simulink model "D53_LKAS_JLU_20200911_1116"  (R2018b)
settings: Solver=ode3  StartTime=0.0  StopTime=10.0  FixedStep=0.01  RelTol=1e-3  EnableMultiTasking=on
model workspace (MAT data in the model file):
  MCOS : class17 (value not decoded)
  MCOS : class17 (value not decoded)
  MCOS : class17 (value not decoded)
  MCOS : class17 (value not decoded)
  MCOS : class17 (value not decoded)
  MCOS : class17 (value not decoded)
  MCOS : class17 (value not decoded)
  MCOS : class17 (value not decoded)
  MCOS : class17 (value not decoded)
  MCOS : class17 (value not decoded)
  MCOS : class17 (value not decoded)
  MCOS : class17 (value not decoded)
  MCOS : class17 (value not decoded)
  MCOS : class17 (value not decoded)
  MCOS : class17 (value not decoded)
  MCOS : class17 (value not decoded)
  MCOS : class17 (value not decoded)
  MCOS : class17 (value not decoded)
  MCOS : class17 (value not decoded)
  MCOS : class17 (value not decoded)
  MCOS : class17 (value not decoded)
  MCOS : class17 (value not decoded)
  MCOS : class17 (value not decoded)
  MCOS : class17 (value not decoded)
  MCOS : class17 (value not decoded)
  MCOS : class17 (value not decoded)
  MCOS : class17 (value not decoded)
  MCOS : class17 (value not decoded)
  MCOS : class17 (value not decoded)
  MCOS : class17 (value not decoded)
  MCOS : class17 (value not decoded)
  MCOS : class17 (value not decoded)
  MCOS : class17 (value not decoded)
  MCOS : class17 (value not decoded)
  MCOS : class17 (value not decoded)
  MCOS : class17 (value not decoded)
  MCOS : class17 (value not decoded)
  MCOS : class17 (value not decoded)
  MCOS : class17 (value not decoded)
  MCOS : class17 (value not decoded)
  MCOS : class17 (value not decoded)
  MCOS : class17 (value not decoded)
  MCOS : class17 (value not decoded)
  MCOS : class17 (value not decoded)
  MCOS : class17 (value not decoded)
  MCOS : class17 (value not decoded)
  MCOS : class17 (value not decoded)
  MCOS : class17 (value not decoded)
  MCOS : class17 (value not decoded)
  MCOS : class17 (value not decoded)
  MCOS : class17 (value not decoded)
  MCOS : class17 (value not decoded)
  MCOS : class17 (value not decoded)
  MCOS : class17 (value not decoded)
  MCOS : class17 (value not decoded)
  MCOS : class17 (value not decoded)
  MCOS : class17 (value not decoded)
  MCOS : class17 (value not decoded)
  MCOS : class17 (value not decoded)
  MCOS : class17 (value not decoded)
  MCOS : class17 (value not decoded)
  MCOS : class17 (value not decoded)
  MCOS : class17 (value not decoded)
  MCOS : class17 (value not decoded)
  MCOS : class17 (value not decoded)
  MCOS : class17 (value not decoded)
  MCOS : class17 (value not decoded)
  MCOS : class17 (value not decoded)
  MCOS : class17 (value not decoded)
  MCOS : class17 (value not decoded)
  MCOS : class17 (value not decoded)
  MCOS : class17 (value not decoded)
  MCOS : class17 (value not decoded)
  MCOS : class17 (value not decoded)
  MCOS : class17 (value not decoded)
  MCOS : class17 (value not decoded)
  MCOS : class17 (value not decoded)
  MCOS : class17 (value not decoded)
  MCOS : class17 (value not decoded)
  MCOS : class17 (value not decoded)
  MCOS : class17 (value not decoded)
  MCOS : class17 (value not decoded)
  MCOS : class17 (value not decoded)
  MCOS : class17 (value not decoded)
  MCOS : class17 (value not decoded)
  MCOS : class17 (value not decoded)
  MCOS : class17 (value not decoded)
  MCOS : class17 (value not decoded)
  MCOS : class17 (value not decoded)
undefined symbols (not defined in the file): LKA_CarWidth, LKA_SampleTime, LKA_StrRatio_C, LKA_Veh2CamL_C, LKA_Veh2CamW_C, LKA_WhlBaseL_C, LL_CompSWA_C, LL_CrvtPrvwT_C, LL_DesDvt_C, LL_DvtComp_C, LL_DvtPrvwT_C, LL_DvtSpdDet_vDvtSpdMin_C, LL_HdAgExT_C, LL_HdAgPrvwT_C, LL_LAccMax_C, LL_LAccRMax_C, LL_LDW_EarliestWarnLine_C, LL_LDW_LatestWarnLine_C, LL_LDWS_SUPPRESS_HEADING, LL_LFClb_TFC_DiffCtlBalance, LL_LFClb_TFC_DiffCtrlMaxSWA, LL_LFClb_TFC_DiffCtrlRatio, LL_LFClb_TFC_facmGainLutGain1_C, LL_LFClb_TFC_facmGainLutGain2_C, LL_LFClb_TFC_facmIntegRatio, LL_LFClb_TFC_facmKlat_C, LL_LFClb_TFC_FfCtlRatio_C, LL_LFClb_TFC_phiIntegCtlMaxSWA_C, LL_LFClb_TFC_tiKlatPrvwT_C, LL_LFClb_TFC_vGainLutVehSpdLwr_C, LL_LFClb_TFC_vGainLutVehSpdUpr_C, LL_LKA_EarliestWarnLine_C, LL_LKA_LatestWarnLine_C, LL_LKAExPrcs_ExitC0Dvt, LL_LKAExPrcs_ExitC0Swt, LL_LKAExPrcs_tiExitTime1, LL_LKAExPrcs_tiExitTime2, LL_LKAExPrcs_tiExitTime3, LL_LKAS_OUT_OF_CONTROL_LAT_VEL, LL_LKAS_OUT_OF_CONTROL_TTLC, LL_LKASWASyn_M0, LL_LKASWASyn_M1, LL_LKASWASyn_M2, LL_LKASWASyn_M3K, LL_LKASWASyn_SWAaddMax, LL_LKASWASyn_T2, LL_LKASWASyn_tiTrqSwaRtTime, LL_LKASWASyn_tiTrqSwaTime, LL_LKASWASyn_TrqMax, LL_LKASWASyn_TrqSwaAddSwt, LL_LKASWASyn_TrqSwaRateDiff, LL_LSpdCompT_C, LL_lStpLngth_C, LL_MAX_DELAY_EPSSTAR_TIME, LL_MAX_DRIVER_TORQUE_DISABLE, LL_MAX_DRIVER_TORQUE_ENABLE, LL_MAX_LANE_WIDTH_DISABLE, LL_MAX_LANE_WIDTH_ENABLE, LL_MAX_LAT_ACC_DISABLE, LL_MAX_LAT_ACC_ENABLE ... (+30)
libraries: simulink x134, canmsglib x52, dspstat3 x3, simulink_extras x1
(part 3 of 18)

== system D53_LKAS_JLU_20200911_1116/Clb/Calibration3 ==
  In1 : Inport
  In2 : Inport  Port=2
  Data Type Conversion{1..10} (10 alike) : DataTypeConversion  OutDataTypeStr=single
  If1 : If  IfExpression=u1 ==21  ElseIfExpressions=u1==22,u1==23,u1==24,u1==25,u1==26,u1==27,u1==28,u1==29,u1==30  ShowElse=off
  Rate Transition{1..3,5..11} (10 alike) : RateTransition  Deterministic=off  OutPortSampleTime=0.01
  Subsystem2 : Subsystem
  Out1 : Outport
  Out2 : Outport  Port=2
  Out3 : Outport  Port=3
  Out4 : Outport  Port=4
  Out5 : Outport  Port=5
  Out6 : Outport  Port=6
  Out7 : Outport  Port=7
  Out8 : Outport  Port=8
  Out9 : Outport  Port=9
  Out10 : Outport  Port=10
  wires:
  If1/3 -> Subsystem2/3(In3)
  If1/6 -> Subsystem2/6(In6)
  If1/2 -> Subsystem2/2(In2)
  If1/5 -> Subsystem2/5(In5)
  If1/9 -> Subsystem2/9(In9)
  If1/4 -> Subsystem2/4(In4)
  If1/1 -> Subsystem2/1(In1)
  If1/7 -> Subsystem2/7(In7)
  If1/8 -> Subsystem2/8(In8)
  If1/10 -> Subsystem2/10(In10)
  In1/1 -> If1/1
  In2/1 -> Subsystem2/11(In11)
  Data Type Conversion3/1 -> Rate Transition3/1
  Data Type Conversion2/1 -> Rate Transition2/1
  Data Type Conversion10/1 -> Rate Transition11/1
  Data Type Conversion5/1 -> Rate Transition6/1
  Rate Transition6/1 -> Out5/1
  Subsystem2/5(Out5) -> Data Type Conversion5/1
  Subsystem2/6(Out6) -> Data Type Conversion6/1
  Subsystem2/10(Out10) -> Data Type Conversion10/1
  Subsystem2/1(Out1) -> Data Type Conversion1/1
  Subsystem2/9(Out9) -> Data Type Conversion9/1
  Subsystem2/7(Out7) -> Data Type Conversion7/1
  Subsystem2/8(Out8) -> Data Type Conversion8/1
  Subsystem2/3(Out3) -> Data Type Conversion3/1
  Subsystem2/4(Out4) -> Data Type Conversion4/1
  Data Type Conversion4/1 -> Rate Transition5/1
  Data Type Conversion8/1 -> Rate Transition9/1
  Data Type Conversion9/1 -> Rate Transition10/1
  Data Type Conversion7/1 -> Rate Transition8/1
  Rate Transition8/1 -> Out7/1
  Rate Transition1/1 -> Out1/1
  Rate Transition2/1 -> Out2/1
  Rate Transition5/1 -> Out4/1
  Rate Transition10/1 -> Out9/1
  Rate Transition11/1 -> Out10/1
  Rate Transition3/1 -> Out3/1
  Subsystem2/2(Out2) -> Data Type Conversion2/1
  Data Type Conversion6/1 -> Rate Transition7/1
  Rate Transition7/1 -> Out6/1
  Data Type Conversion1/1 -> Rate Transition1/1
  Rate Transition9/1 -> Out8/1

== system D53_LKAS_JLU_20200911_1116/Clb/Subsystem1 ==
  CAN Unpack : canmsglib/CAN Unpack  MsgList=(none)  MsgName=CAN Msg  MsgIDType=Extended (29-bit identifier)  MsgIdentifier=120534787  MsgLength=8  SignalInfo=Serial number$0$8$1$2$1$0$1$0$-Inf$Inf$#index$8$8$1$2$1$0$1$-100$-Inf$Inf$#coefficient$16$32$1$2$1$0$0.000001$-10$-Inf$Inf$#  NSignals=3  IDPort=off  TimestampPort=off  ErrorPort=off  RemotePort=off  LengthPort=off  StatusPort=off  StartBits=str2num('[int32(0);int32(8);int32(16)]')  SignalSizes=str2num('[int32(8);int32(8);int32(32)]')  ByteOrders=str2num('[int32(1);int32(1);int32(1)]')  DataTypes=str2num('[int32(2);int32(2);int32(2)]')  MultiplexTypes=str2num('[int32(1);int32(1);int32(1)]')  MultiplexValues=str2num('[double(0);double(0);double(0)]')  Factors=str2num('[double(1);double(1);double(0.000001)]')  Offsets=str2num('[double(0);double(-100);double(-10)]')  Minimums=str2num('[double(-Inf);double(-Inf);double(-Inf)]')  Maximums=str2num('[double(Inf);double(Inf);double(Inf)]')  ApplyMinMax=off
      settings: SourceProductName=Simulink Real-Time  SourceProductBaseCode=XP
  S-Function2 : S-Function  FunctionName=CAN_Rec_P  Parameters=uint8(Module-1),uint32(ID),uint8(Frameformat-1),uint8(Newflag),uint8(FIFO),double(sampletime)  SFunctionDeploymentMode=off  EnableBusSupport=off  mask(CAN_receive){Module=CAN_0, ID=120534787, Frameformat=Extended (29-bit identifier), Newflag=on, FIFO=off, sampletime=0.01}
      mask prompts: Module "CAN Port:"; ID "CAN Frame ID:"; Frameformat "CAN Frame Format:"; FIFO "Overflow flag"
      mask init:
      | maskdisplay = canrecicon(Module,ID,Frameformat,Newflag,FIFO);
      | set_param(gcb, 'MaskDisplay', maskdisplay);
      mask TypeOptions Module: CAN_0 | CAN_1 | CAN_2 | CAN_3
      mask TypeOptions Frameformat: Standard (11-bit identifier) | Extended (29-bit identifier)
      mask Display: color('blue');text(0.98,0.9,'MPC5675K','horizontalAlignment','right');color('black');text(0.5,0.6,'FlexCAN_0 Receive','horizontalAlignment','center');text(0.5,0.35,'Extended ID:120534787','horizontalAlignment','center');port_label('output',1,'New_Flag');port_label('output',2,'CAN_Msg');
  Out1 : Outport
  Out2 : Outport  Port=2
  Out3 : Outport  Port=3
  wires:
  S-Function2/2 -> CAN Unpack/1
  CAN Unpack/1 -> Out1/1
  CAN Unpack/2 -> Out2/1
  CAN Unpack/3 -> Out3/1

== system D53_LKAS_JLU_20200911_1116/Clb/Subsystem5 ==
  In1 : Inport
  In2 : Inport  Port=2
  Constant : Constant  Value=10
  Data Type Conversion1 : DataTypeConversion  OutDataTypeStr=single
  Data Type Conversion3 : DataTypeConversion  OutDataTypeStr=single
  Divide : Product  Inputs=**
  Fcn : Fcn  Expr=pow(u(1),u(2))
  Mux : Mux  Inputs=2
  Out1 : Outport
  wires:
  Mux/1 -> Fcn/1
  Fcn/1 -> Divide/1
  In2/1 -> Divide/2
  Divide/1 -> Out1/1
  In1/1 -> Data Type Conversion1/1
  Data Type Conversion1/1 -> Mux/2
  Data Type Conversion3/1 -> Mux/1
  Constant/1 -> Data Type Conversion3/1

== system D53_LKAS_JLU_20200911_1116/LL/Fault_Diagnostic ==
  bsInInfo : Inport
  Bus Creator : BusCreator  Inputs=2
  Bus Creator1 : BusCreator  Inputs=12
  Bus Selector3 : BusSelector  OutputSignals=DTC_Indicator.LKAS_BSWDTC_Status
  Bus Selector4 : BusSelector  OutputSignals=bsVehMovInfo.ESC_VehSpd_Valid,bsEPSInfo.EPS_LKA_State,bsEPSInfo.EPS_Error_State,bsEPSInfo.SAS_Clb_State,bsEPSInfo.SAS_Trim_State,bsSWAInfo.SWS_Fault_Code,bsSWAInfo.SAS_In_Status,bsPTState.TCU_ActualGear,bsEPSInfo.EPS_TrqLim_State,bsEPSInfo.EPS_Trq_State,bsVehMovInfo.ESC_LatAcc_Valid,bsVehMovInfo.ESC_YawRate_Valid,bsVehMovInfo.ESC_LonAcc_Valid
  Compare To Constant26 : simulink/Logic and Bit Operations/Compare To Constant  relop=~=  const=1  OutDataTypeStr=boolean
  Compare To Constant27 : simulink/Logic and Bit Operations/Compare To Constant  relop===  const=4  OutDataTypeStr=boolean
  Compare To Constant{28,30,36..39} (6 alike) : simulink/Logic and Bit Operations/Compare To Constant  relop===  const=1  OutDataTypeStr=boolean
  Compare To Constant29 : simulink/Logic and Bit Operations/Compare To Constant  relop===  const=0  OutDataTypeStr=boolean
  Compare To Constant31 : simulink/Logic and Bit Operations/Compare To Constant  relop===  const=2  OutDataTypeStr=boolean
  Compare To Constant32 : simulink/Logic and Bit Operations/Compare To Constant  relop=~=  const=0  OutDataTypeStr=boolean
  Compare To Constant33 : simulink/Logic and Bit Operations/Compare To Constant  relop=~=  const=1  OutDataTypeStr=boolean
  Compare To Constant34 : simulink/Logic and Bit Operations/Compare To Constant  relop=>  const=3  OutDataTypeStr=boolean
  Compare To Constant35 : simulink/Logic and Bit Operations/Compare To Constant  relop===  const=0  OutDataTypeStr=boolean
  Logical Operator5 : Logic  Operator=OR  AllPortsSameDT=off  OutDataTypeStr=boolean
  Logical Operator6 : Logic  Operator=OR  AllPortsSameDT=off  OutDataTypeStr=boolean
  bsSignalFault : Outport
  wires:
  Logical Operator6/1 -> Bus Creator1/6  "Event_FaulSWS"
  Logical Operator5/1 -> Bus Creator1/3  "Event_FaulETATDA"
  Compare To Constant27/1 -> Bus Creator1/2  "Event_FaulEPSLKASt"
  Bus Creator1/1 -> Bus Creator/2  "LKAS_ASWDTC_Status"
  Compare To Constant39/1 -> Bus Creator1/12  "Event_FaulLonAcc"
  Compare To Constant38/1 -> Bus Creator1/11  "Event_FaulYawRate"
  Compare To Constant37/1 -> Bus Creator1/10  "Event_FaulLatAcc"
  Compare To Constant36/1 -> Bus Creator1/9  "Event_FaulEPSTrqSt"
  Compare To Constant34/1 -> Bus Creator1/7  "Event_FaulTCUGear"
  Compare To Constant35/1 -> Bus Creator1/8  "Event_FaulTrqLim"
  Compare To Constant33/1 -> Logical Operator6/2
  Compare To Constant32/1 -> Logical Operator6/1
  Bus Selector4/3 -> Compare To Constant28/1, Compare To Constant31/1  "<EPS_Error_State>"
  Compare To Constant28/1 -> Logical Operator5/1
  Compare To Constant31/1 -> Logical Operator5/2
  Compare To Constant30/1 -> Bus Creator1/5  "Event_FaulSASTrim"
  Bus Selector4/13 -> Compare To Constant39/1  "<ESC_LonAcc_Valid>"
  Bus Selector4/12 -> Compare To Constant38/1  "<ESC_YawRate_Valid>"
  Bus Selector4/11 -> Compare To Constant37/1  "<ESC_LatAcc_Valid>"
  Bus Selector4/10 -> Compare To Constant36/1  "<EPS_Trq_State>"
  Bus Selector4/9 -> Compare To Constant35/1  "<EPS_TrqLim_State>"
  Bus Selector4/8 -> Compare To Constant34/1  "<TCU_ActualGear>"
  Bus Selector4/7 -> Compare To Constant33/1  "<SAS_In_Status>"
  Bus Selector4/6 -> Compare To Constant32/1  "<SWS_Fault_Code>"
  Bus Selector4/5 -> Compare To Constant30/1  "<SAS_Trim_State>"
  Compare To Constant29/1 -> Bus Creator1/4  "Event_FaulSASClb"
  Bus Selector4/4 -> Compare To Constant29/1  "<SAS_Clb_State>"
  Bus Selector4/2 -> Compare To Constant27/1  "<EPS_LKA_State>"
  Compare To Constant26/1 -> Bus Creator1/1  "Event_FaulVehSpeed"
  Bus Selector4/1 -> Compare To Constant26/1  "<ESC_VehSpd_Valid>"
  bsInInfo/1 -> Bus Selector3/1, Bus Selector4/1
  Bus Selector3/1 -> Bus Creator/1  "<LKAS_BSWDTC_Status>"
  Bus Creator/1 -> bsSignalFault/1

== system D53_LKAS_JLU_20200911_1116/LL/Human Machine Interface (HMI) ==
  HMI_stDACmode : Inport
  HMI_LDWWarn : Inport  Port=2
  HMI_LKA_STATE : Inport  Port=3
  HMI_LDW_STATE : Inport  Port=4
  HMI_R0_Quality : Inport  Port=5
  HMI_L0_Quality : Inport  Port=6
  HMI_EPSInfo : Inport  Port=7
  HMI_camera_common_fault : Inport  Port=8
  HMI_Front_Camera_Blocked : Inport  Port=9
  HMI_stFaultCSyn : Inport  Port=10
  Bus Creator2 : BusCreator  Inputs=7
  Cast To Single{,1..6} (7 alike) : DataTypeConversion  OutDataTypeStr=uint8
  HMI_Popup_Status : MATLAB Function  TreatAsAtomicUnit=on
  Hands_off_warning : MATLAB Function  TreatAsAtomicUnit=on
  LDW_Flag : MATLAB Function  TreatAsAtomicUnit=on
  LDW_Status_Display : MATLAB Function  TreatAsAtomicUnit=on
  LKA_Status_Display : MATLAB Function  TreatAsAtomicUnit=on
  LKA_action_indication : MATLAB Function  TreatAsAtomicUnit=on
  Subsystem : Subsystem
  Vehicle_Lane_Display : MATLAB Function  TreatAsAtomicUnit=on
  HMI_LDWLKA : Outport
  wires:
  HMI_LDWWarn/1 -> LDW_Flag/3(HMI_LDWWarnInfo)
  Subsystem/2(HandsOff15s) -> Hands_off_warning/1(HandsOff)
  Subsystem/1(HandsOff10s) -> HMI_Popup_Status/3(HandsOff)
  HMI_EPSInfo/1 -> Subsystem/2(EPSInfo)  "HMI_EPSInfo"
  Cast To Single6/1 -> Bus Creator2/7  "HMI_Popup_Status"
  Cast To Single5/1 -> Bus Creator2/6  "LKA_action_indication"
  Cast To Single4/1 -> Bus Creator2/5  "Hands_off_warning"
  Cast To Single3/1 -> Bus Creator2/4  "LDW_Flag"
  Cast To Single2/1 -> Bus Creator2/3  "LKA_Status_Display"
  Cast To Single1/1 -> Bus Creator2/2  "LDW_Status_Display"
  Cast To Single/1 -> Bus Creator2/1  "Vehicle_Lane_Display"
  Vehicle_Lane_Display/1(Vehicle_Lane_Display) -> Cast To Single/1  "Vehicle_Lane_Display"
  LKA_action_indication/1(LKA_action_indication) -> Cast To Single5/1  "LKA_action_indication"
  HMI_camera_common_fault/1 -> HMI_Popup_Status/4(camera_common_fault)  "HMI_camera_common_fault"
  HMI_R0_Quality/1 -> Vehicle_Lane_Display/4(R0_Quality)  "HMI_R0_Quality"
  HMI_Front_Camera_Blocked/1 -> HMI_Popup_Status/5(Front_Camera_Blocked)  "HMI_Front_Camera_Blocked"
  LDW_Flag/1(LDW_Flag) -> Cast To Single3/1  "LDW_Flag"
  HMI_stDACmode/1 -> LKA_Status_Display/1(stDACmode), LDW_Flag/1(HMI_stDACmode), LKA_action_indication/1(stDACmode), HMI_Popup_Status/1(stDACmode), LDW_Status_Display/1(stDACmode), Vehicle_Lane_Display/1(stDACmode)  "HMI_stDACmode"
  LKA_Status_Display/1(LKA_Status_Display) -> Cast To Single2/1  "LKA_Status_Display"
  HMI_Popup_Status/1(HMI_Popup_Status) -> Cast To Single6/1  "HMI_Popup_Status"
  HMI_L0_Quality/1 -> Vehicle_Lane_Display/5(L0_Quality)  "HMI_L0_Quality"
  Bus Creator2/1 -> HMI_LDWLKA/1
  HMI_stFaultCSyn/1 -> HMI_Popup_Status/6(stFaultCSyn)  "HMI_stFaultCSyn"
  LDW_Status_Display/1(LDW_Status_Display) -> Cast To Single1/1  "LDW_Status_Display"
  Hands_off_warning/1(Hands_off_warning) -> Cast To Single4/1  "Hands_off_warning"
  HMI_LDW_STATE/1 -> LDW_Status_Display/2(LDW_STATE), Vehicle_Lane_Display/3(LDW_STATE), Subsystem/1(LDW_STATE)  "HMI_LDW_STATE"
  HMI_LKA_STATE/1 -> LKA_action_indication/2(LKA_STATE), HMI_Popup_Status/2(LKA_STATE), LDW_Flag/2(HMI_LKA_STATE), LKA_Status_Display/2(LKA_STATE), Vehicle_Lane_Display/2(LKA_STATE)  "HMI_LKA_STATE"

== system D53_LKAS_JLU_20200911_1116/LL/LL Inputs Mapping ==
  bsInInfo : Inport
  Bus Creator : BusCreator  Inputs=7
  Bus Selector : BusSelector  OutputSignals=bsMP5Info,bsLaneInfo,bsEPSInfo,bsVehMovInfo,bsSWAInfo,bsBCMInfo,bsPTState
  bsBCMInfo : Subsystem
  bsEPSInfo : Subsystem
  bsLaneInfo : Subsystem
  bsMP5Info : Subsystem
  bsPTState : Subsystem
  bsSWAInfo : Subsystem
  bsVehMovInfo : Subsystem
  bsInfo : Outport
  wires:
  bsInInfo/1 -> Bus Selector/1
  Bus Creator/1 -> bsInfo/1
  Bus Selector/2 -> bsLaneInfo/1(bsLaneInfoIn)  "<bsLaneInfo>"
  Bus Selector/3 -> bsEPSInfo/1(bsEPSInfoIn)  "<bsEPSInfo>"
  bsEPSInfo/1(bsEPSInfoOut) -> Bus Creator/3  "bsEPSInfo"
  Bus Selector/4 -> bsVehMovInfo/1(bsVehMovInfoIn)  "<bsVehMovInfo>"
  bsVehMovInfo/1(bsVehMovInfoOut) -> Bus Creator/4  "bsVehMovInfo"
  Bus Selector/5 -> bsSWAInfo/1(bsSWAInfoIn)  "<bsSWAInfo>"
  Bus Selector/6 -> bsBCMInfo/1(bsBCMInfoIn)  "<bsBCMInfo>"
  Bus Selector/1 -> bsMP5Info/1(bsMP5InfoIn)  "<bsMP5Info>"
  bsMP5Info/1(bsMP5InfoOut) -> Bus Creator/1  "bsMP5Info"
  bsBCMInfo/1(bsBCMInfoOut) -> Bus Creator/6  "bsBCMInfo"
  Bus Selector/7 -> bsPTState/1(bsPTStateIn)  "<bsPTState>"
  bsPTState/1(bsPTStateOut) -> Bus Creator/7  "bsPTState"
  bsLaneInfo/1(bsLaneInfoOut) -> Bus Creator/2  "bsLaneInfo"
  bsSWAInfo/1(bsSWAInfoOut) -> Bus Creator/5  "bsSWAInfo"

== system D53_LKAS_JLU_20200911_1116/LL/LL Output (LLOut) ==
  LLOut_bsLLState : Inport
  LLOut_phiSWACmd : Inport  Port=2
  LLOut_bsLLHMI : Inport  Port=3
  LLOut_M : Inport  Port=4
  Bus Creator : BusCreator  Inputs=15
  Bus Selector1 : BusSelector  OutputSignals=LKA_State,DACMode
  Bus Selector2 : BusSelector  OutputSignals=Vehicle_Lane_Display,LDW_Status_Display,LKA_Status_Display,LDW_Flag,Hands_off_warning,LKA_action_indication,HMI_Popup_Status
  Cast To Single : DataTypeConversion  OutDataTypeStr=single
  Cast To Single{2,4..15} (13 alike) : DataTypeConversion  OutDataTypeStr=uint8
  Cast To Single3 : DataTypeConversion  OutDataTypeStr=single
  Compare To Constant : simulink/Logic and Bit Operations/Compare To Constant  relop===  const=4  OutDataTypeStr=boolean
  Compare To Constant1 : simulink/Logic and Bit Operations/Compare To Constant  relop=>  const=0  OutDataTypeStr=boolean
  Constant : Constant  Value=0  OutDataTypeStr=uint8
  Constant1 : Constant  OutDataTypeStr=uint8
  Constant15 : Constant  Value=0  OutDataTypeStr=uint16
  Constant2 : Constant  Value=2  OutDataTypeStr=uint8
  Constant25 : Constant  Value=0  OutDataTypeStr=uint8
  Constant26 : Constant  Value=0  OutDataTypeStr=uint8
  Constant3 : Constant  Value=3  OutDataTypeStr=uint8
  Constant4 : Constant  Value=4  OutDataTypeStr=uint8
  Constant5 : Constant  Value=4  OutDataTypeStr=uint8
  Constant6 : Constant  Value=5  OutDataTypeStr=uint8
  Constant7 : Constant  Value=0  OutDataTypeStr=single
  Multiport Switch : MultiPortSwitch  DataPortOrder=Zero-based contiguous  Inputs=7  zeroidx=on
  Switch : Switch  Criteria=u2 > Threshold
  LL_bsLLOut : Outport
  wires:
  Cast To Single7/1 -> Bus Creator/7  "LKA_action_indication"
  Bus Selector2/7 -> [HMI_Popup_Status]  "<HMI_Popup_Status>"
  Compare To Constant/1 -> Switch/2
  [Vehicle_Lane_Display] -> Cast To Single12/1  "Vehicle_Lane_Display"
  Constant15/1 -> Cast To Single4/1  "Permit_to_know_if_LKA_or_LPA3F2"
  [LDW_Flag] -> Cast To Single5/1  "LDW_Flag"
  [Coefficient_toregulate_EPS] -> Cast To Single3/1  "Coefficient_toregulate_EPS"
  [LKA_action_indication] -> Cast To Single7/1  "LKA_action_indication"
  Constant6/1 -> Multiport Switch/8
  Cast To Single5/1 -> Bus Creator/5  "LDW_Flag"
  [HMI_Popup_Status] -> Cast To Single9/1  "HMI_Popup_Status"
  Bus Selector1/1 -> Multiport Switch/1  "<LKA_State>"
  [LKA_Status_Display] -> Cast To Single8/1  "LKA_Status_Display"
  Bus Selector2/4 -> [LDW_Flag]  "<LDW_Flag>"
  LLOut_phiSWACmd/1 -> Cast To Single/1  "LMS_phiSWACmd"
  Bus Selector2/3 -> [LKA_Status_Display]  "<LKA_Status_Display>"
  Cast To Single/1 -> Bus Creator/1  "LMS_phiSWACmd"
  [LDW_Status_Display] -> Cast To Single6/1  "LDW_Status_Display"
  [LKA_Switch_State] -> Cast To Single10/1  "LKA_Switch_State"
  [Hands_off_warning] -> Cast To Single11/1  "Hands_off_warning"
  Constant26/1 -> Cast To Single15/1  "TJA_status_icon"
  Cast To Single8/1 -> Bus Creator/8  "LKA_Status_Display"
  Cast To Single4/1 -> Bus Creator/4  "Permit_to_know_if_LKA_or_LPA3F2"
  Cast To Single10/1 -> Bus Creator/10  "LKA_Switch_State"
  Bus Selector1/2 -> Compare To Constant1/1, [LKA_Mode_from_Camera]  "<DACMode>"
  Constant2/1 -> Multiport Switch/4
  Cast To Single2/1 -> Bus Creator/2  "EPS_State_Ctl"
  Bus Creator/1 -> LL_bsLLOut/1  "LL_bsLLOut"
  Cast To Single14/1 -> Bus Creator/14  "TJA_HMI_Txt_Disp"
  Cast To Single3/1 -> Bus Creator/3  "Coefficient_toregulate_EPS"
  Constant3/1 -> Multiport Switch/5
  Bus Selector2/5 -> [Hands_off_warning]  "<Hands_off_warning>"
  Multiport Switch/1 -> Compare To Constant/1, [EPS_State_Ctl]  "EPS_State_Ctl"
  Switch/1 -> [Coefficient_toregulate_EPS]  "Coefficient_toregulate_EPS"
  Constant7/1 -> Switch/3
  Cast To Single6/1 -> Bus Creator/6  "LDW_Status_Display"
  Cast To Single12/1 -> Bus Creator/12  "Vehicle_Lane_Display"
  [LKA_Mode_from_Camera] -> Cast To Single13/1  "LKA_Mode_from_Camera"
  [EPS_State_Ctl] -> Cast To Single2/1  "EPS_State_Ctl"
  LLOut_bsLLHMI/1 -> Bus Selector2/1
  Bus Selector2/1 -> [Vehicle_Lane_Display]  "<Vehicle_Lane_Display>"
  Constant1/1 -> Multiport Switch/3
  LLOut_bsLLState/1 -> Bus Selector1/1
  Compare To Constant1/1 -> [LKA_Switch_State]
  Cast To Single15/1 -> Bus Creator/15  "TJA_status_icon"
  Bus Selector2/6 -> [LKA_action_indication]  "<LKA_action_indication>"
  Constant4/1 -> Multiport Switch/6
  Cast To Single9/1 -> Bus Creator/9  "HMI_Popup_Status"
  Bus Selector2/2 -> [LDW_Status_Display]  "<LDW_Status_Display>"
  LLOut_M/1 -> Switch/1
  Constant25/1 -> Cast To Single14/1  "TJA_HMI_Txt_Disp"
  Cast To Single11/1 -> Bus Creator/11  "Hands_off_warning"
  Cast To Single13/1 -> Bus Creator/13  "LKA_Mode_from_Camera"
  Constant5/1 -> Multiport Switch/7
  Constant/1 -> Multiport Switch/2

== system D53_LKAS_JLU_20200911_1116/LL/LLOn ==
  stDACMode : Inport
  bsInInfo : Inport  Port=2
  bsLLClb : Inport  Port=3
  bsSignalFault : Inport  Port=4
  states : EnablePort  StatesWhenEnabling=reset
      settings: AttributesFormatString=states = %<StatesWhenEnabling>
  Bus Selector : BusSelector  OutputSignals=bsLLSMConClb,bsLDWClb,bsLKAClb,bsConstantClb
  LDW : Subsystem  Description=|  TreatAsAtomicUnit=on
      | Block Name: Lane Departure Warning
      | Ab.: LDW
      | No.: 1.3.0.0
      | Rev: 0.0.1
      | Update Date: 19-3-26
  LKA : Subsystem  Description=|  TreatAsAtomicUnit=on
      | Block Name: Lane Keeping Assistance
      | Ab.: LKA
      | No.: 1.2.0.0
      | Rev: 0.0.1
      | Update Date: 19-5-13
  LKA Input Processing (LKAInP) : Subsystem
  LL State Determination (LLStateDet) : Subsystem
  LL_Mon : Subsystem
  bsLLState : Outport  OutputWhenDisabled=reset  InitialOutput=0
  LDW_Flag : Outport  Port=2
  phiSWACmd : Outport  Port=3  OutputWhenDisabled=reset  InitialOutput=0
  M : Outport  Port=4  OutputWhenDisabled=reset  InitialOutput=0
  LLMon : Outport  Port=5
  tag scope: LLClb_bsConstantClb=global, LLClb_bsLLSMConClb=global
  wires:
  LL_Mon/1(LLMon) -> LLMon/1
  [LKAMon] -> LL_Mon/1(LKAMon)
  LKA/4(LKAMon) -> [LKAMon]
  LKA/3(LKA_M) -> M/1  "OutputM"
  bsSignalFault/1 -> LL State Determination (LLStateDet)/6(LLStateDet_SignalFault)
  LKA/1(LKA_ExitFlg) -> [ExitFlg]
  LKA/2(LKA_phiSWACmd) -> phiSWACmd/1  "OutputSWACmd"
  [LLClb_bsConstantClb] -> LKA/4(LKA_bsConstantClb)
  Bus Selector/4 -> [LLClb_bsConstantClb]  "<bsConstantClb>"
  [ExitFlg] -> LL State Determination (LLStateDet)/5(LLStateDet_stExitFlg)
  bsInInfo/1 -> LDW/2(LDW_bsInInfoSyn), LKA/1(LKA_bsInInfoSyn), LL State Determination (LLStateDet)/2(LLStateDet_bsInInfoSyn), LKA Input Processing (LKAInP)/2(LKAInP_bsInInfoSyn)
  LDW/1(LDW_Flag) -> LDW_Flag/1  "LDW_Flag"
  LL State Determination (LLStateDet)/3(LLStateDet_stLKAActvFlg) -> LKA/Enable, [ActFlg]
  Bus Selector/2 -> [LLClb_bsLDWClb]  "<bsLDWClb>"
  Bus Selector/3 -> [LLClb_bsLKAClb]  "<bsLKAClb>"
  stDACMode/1 -> LL State Determination (LLStateDet)/1(LLStateDet_stDACMode)
  Bus Selector/1 -> [LLClb_bsLLSMConClb]  "<bsLLSMConClb>"
  [LLClb_bsLKAClb] -> LKA/3(LKA_bsLKAClb)
  bsLLClb/1 -> Bus Selector/1
  LKA Input Processing (LKAInP)/1(LKAInP_bsLKAInPInfo) -> LL State Determination (LLStateDet)/3(LLStateDet_bsLKAInPInfo), LKA/2(LKA_bsLKAInPInfo)
  [LLClb_bsLDWClb] -> LDW/3(LDW_bsLDWClb)
  LL State Determination (LLStateDet)/1(LLStateDet_bsLLState) -> bsLLState/1
  [LLClb_bsLKAClb] -> LKA Input Processing (LKAInP)/3(LKAInP_bsLKAClb)
  [LLClb_bsLLSMConClb] -> LL State Determination (LLStateDet)/4(LLStateDet_bsLLSMConClb)
  LL State Determination (LLStateDet)/2(LLStateDet_stLDWActvFlg) -> LDW/1(LDW_stLDWActvFlg), LDW/Enable
  [ActFlg] -> LKA Input Processing (LKAInP)/1(LKAInP_stLKAActvFlg)

== system D53_LKAS_JLU_20200911_1116/LL/Subsystem ==
  bsInfo : Inport
  Bus Selector : BusSelector  OutputSignals=bsMP5Info.LKA_Main_Switch,bsMP5Info.LKA_Mode
  On : Outport  OutDataTypeStr=uint8
  Mode : Outport  Port=2  OutDataTypeStr=uint8
  wires:
  Bus Selector/1 -> On/1  "<LKA_Main_Switch>"
  bsInfo/1 -> Bus Selector/1
  Bus Selector/2 -> Mode/1  "<LKA_Mode>"

== system D53_LKAS_JLU_20200911_1116/LLClb/ConstantClb ==
  Bus Creator : BusCreator  Inputs=6
  Data Type Conversion{2..4,6,13,22} (6 alike) : DataTypeConversion  OutDataTypeStr=single
  LKA_CarWidth=1.8 : Constant  Value=LKA_CarWidth
  LKA_SampleTime=0.01 : Constant  Value=LKA_SampleTime  OutDataTypeStr=single
  LKA_StrRatio_C=15.3 : Constant  Value=LKA_StrRatio_C
  LKA_Veh2CamL_C=1.56 : Constant  Value=LKA_Veh2CamL_C
  LKA_Veh2CamW_C=0.9 : Constant  Value=LKA_Veh2CamW_C  OutDataTypeStr=single
  LKA_WhlBaseL_C=2.65 : Constant  Value=LKA_WhlBaseL_C
  Switch{,1..3,11,19} (6 alike) : Switch  Criteria=u2 ~= 0  OutDataTypeStr=single
  ConstantClb : Outport
  wires:
  LKA_Veh2CamW_C=0.9/1 -> Switch/3  "LKA_Veh2CamW_C"
  Data Type Conversion13/1 -> Switch/1, Switch/2
  Data Type Conversion2/1 -> Switch1/1, Switch1/2
  LKA_Veh2CamL_C=1.56/1 -> Switch1/3  "LKA_Veh2CamL_C"
  LKA_WhlBaseL_C=2.65/1 -> Switch2/3  "LKA_WhlBaseL_C"
  Data Type Conversion4/1 -> Switch2/1, Switch2/2
  Data Type Conversion6/1 -> Switch3/1, Switch3/2
  LKA_StrRatio_C=15.3/1 -> Switch3/3  "LKA_StrRatio_C"
  Data Type Conversion22/1 -> Switch11/1, Switch11/2
  LKA_CarWidth=1.8/1 -> Switch11/3  "LKA_CarWidth"
  Bus Creator/1 -> ConstantClb/1
  Switch3/1 -> Bus Creator/5  "LKA_StrRatio_C"
  Switch11/1 -> Bus Creator/6  "LKA_CarWidth"
  Switch1/1 -> Bus Creator/3  "LKA_Veh2CamL_C"
  Switch/1 -> Bus Creator/2  "LKA_Veh2CamW_C"
  Switch2/1 -> Bus Creator/4  "LKA_WhlBaseL_C"
  Switch19/1 -> Bus Creator/1  "LKA_SampleTime"
  Data Type Conversion3/1 -> Switch19/2, Switch19/1
  LKA_SampleTime=0.01/1 -> Switch19/3  "LKA_SampleTime"

== system D53_LKAS_JLU_20200911_1116/LLClb/LDWClb ==
  Bus Creator : BusCreator  Inputs=1
  Data Type Conversion6 : DataTypeConversion  OutDataTypeStr=single
  LL_LDWS_SUPPRESS_HEADING=2 : Constant  Value=LL_LDWS_SUPPRESS_HEADING  OutDataTypeStr=single
  Switch2 : Switch  Criteria=u2 ~= 0  OutDataTypeStr=single
  LDWClb : Outport
  wires:
  Bus Creator/1 -> LDWClb/1
  Switch2/1 -> Bus Creator/1  "LL_LDWS_SUPPRESS_HEADING"
  LL_LDWS_SUPPRESS_HEADING=2/1 -> Switch2/3
  Data Type Conversion6/1 -> Switch2/1, Switch2/2

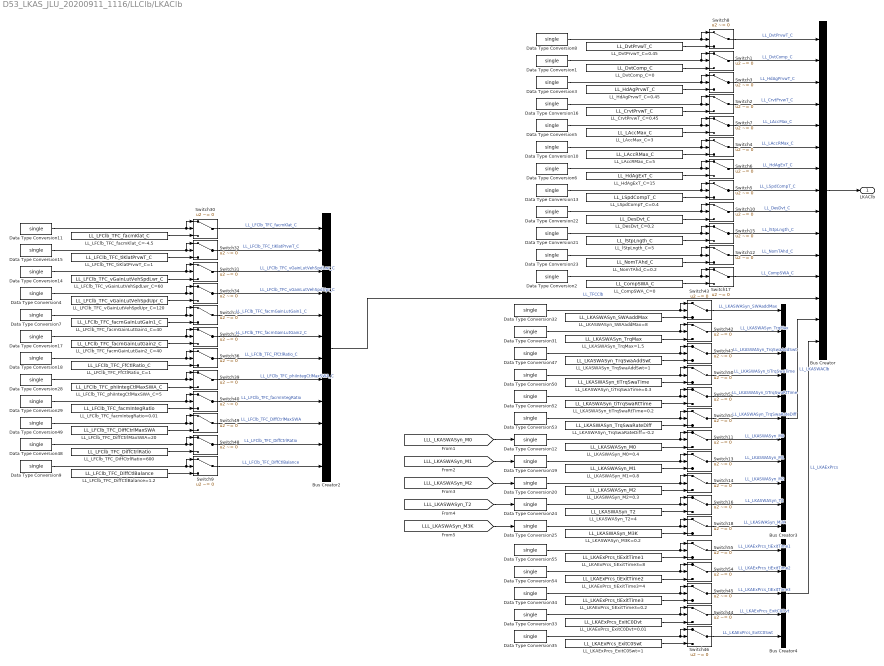
== system D53_LKAS_JLU_20200911_1116/LLClb/LKAClb ==
  Bus Creator : BusCreator  Inputs=15
  Bus Creator2 : BusCreator  Inputs=12
  Bus Creator3 : BusCreator  Inputs=11
  Bus Creator4 : BusCreator  Inputs=5
  Data Type Conversion{1..25,28..29,31..35,47..50,52..55} (40 alike) : DataTypeConversion  OutDataTypeStr=single
  LL_CompSWA_C=0 : Constant  Value=LL_CompSWA_C  OutDataTypeStr=single
  LL_CrvtPrvwT_C=0.45 : Constant  Value=LL_CrvtPrvwT_C  OutDataTypeStr=single
  LL_DesDvt_C=0.2 : Constant  Value=LL_DesDvt_C  OutDataTypeStr=single
  LL_DvtComp_C=0 : Constant  Value=LL_DvtComp_C  OutDataTypeStr=single
  LL_DvtPrvwT_C=0.45 : Constant  Value=LL_DvtPrvwT_C  OutDataTypeStr=single
  LL_HdAgExT_C=15 : Constant  Value=LL_HdAgExT_C  OutDataTypeStr=single
  LL_HdAgPrvwT_C=0.45 : Constant  Value=LL_HdAgPrvwT_C  OutDataTypeStr=single
  LL_LAccMax_C=3 : Constant  Value=LL_LAccMax_C  OutDataTypeStr=single
  LL_LAccRMax_C=5 : Constant  Value=LL_LAccRMax_C  OutDataTypeStr=single
  LL_LFClb_TFC_DiffCtlBalance=1.2 : Constant  Value=LL_LFClb_TFC_DiffCtlBalance  OutDataTypeStr=single
  LL_LFClb_TFC_DiffCtrlMaxSWA=20 : Constant  Value=LL_LFClb_TFC_DiffCtrlMaxSWA  OutDataTypeStr=single
  LL_LFClb_TFC_DiffCtrlRatio=600 : Constant  Value=LL_LFClb_TFC_DiffCtrlRatio  OutDataTypeStr=single
  LL_LFClb_TFC_FfCtlRatio_C=1 : Constant  Value=LL_LFClb_TFC_FfCtlRatio_C  OutDataTypeStr=single
  LL_LFClb_TFC_facmGainLutGain1_C=40 : Constant  Value=LL_LFClb_TFC_facmGainLutGain1_C  OutDataTypeStr=single
  LL_LFClb_TFC_facmGainLutGain2_C=40 : Constant  Value=LL_LFClb_TFC_facmGainLutGain2_C  OutDataTypeStr=single
  LL_LFClb_TFC_facmIntegRatio=0.01 : Constant  Value=LL_LFClb_TFC_facmIntegRatio  OutDataTypeStr=single
  LL_LFClb_TFC_facmKlat_C=-4.5 : Constant  Value=LL_LFClb_TFC_facmKlat_C  OutDataTypeStr=single
  LL_LFClb_TFC_phiIntegCtlMaxSWA_C=5 : Constant  Value=LL_LFClb_TFC_phiIntegCtlMaxSWA_C  OutDataTypeStr=single
  LL_LFClb_TFC_tiKlatPrvwT_C=1 : Constant  Value=LL_LFClb_TFC_tiKlatPrvwT_C  OutDataTypeStr=single
  LL_LFClb_TFC_vGainLutVehSpdLwr_C=60 : Constant  Value=LL_LFClb_TFC_vGainLutVehSpdLwr_C  OutDataTypeStr=single
  LL_LFClb_TFC_vGainLutVehSpdUpr_C=120 : Constant  Value=LL_LFClb_TFC_vGainLutVehSpdUpr_C  OutDataTypeStr=single
  LL_LKAExPrcs_ExitC0Dvt=0.01 : Constant  Value=LL_LKAExPrcs_ExitC0Dvt  OutDataTypeStr=single
  LL_LKAExPrcs_ExitC0Swt=1 : Constant  Value=LL_LKAExPrcs_ExitC0Swt  OutDataTypeStr=single
  LL_LKAExPrcs_tiExitTime3=0.2 : Constant  Value=LL_LKAExPrcs_tiExitTime3  OutDataTypeStr=single
  LL_LKAExPrcs_tiExitTime3=4 : Constant  Value=LL_LKAExPrcs_tiExitTime2  OutDataTypeStr=single
  LL_LKAExPrcs_tiExitTime3=8 : Constant  Value=LL_LKAExPrcs_tiExitTime1  OutDataTypeStr=single
  LL_LKASWASyn_M0=0.4 : Constant  Value=LL_LKASWASyn_M0  OutDataTypeStr=single
  LL_LKASWASyn_M1=0.8 : Constant  Value=LL_LKASWASyn_M1  OutDataTypeStr=single
  LL_LKASWASyn_M2=0.3 : Constant  Value=LL_LKASWASyn_M2  OutDataTypeStr=single
  LL_LKASWASyn_M3K=0.2 : Constant  Value=LL_LKASWASyn_M3K  OutDataTypeStr=single
  LL_LKASWASyn_SWAaddMax=8 : Constant  Value=LL_LKASWASyn_SWAaddMax  OutDataTypeStr=single
  LL_LKASWASyn_T2=4 : Constant  Value=LL_LKASWASyn_T2  OutDataTypeStr=single
  LL_LKASWASyn_TrqMax=1.5 : Constant  Value=LL_LKASWASyn_TrqMax  OutDataTypeStr=single
  LL_LKASWASyn_TrqSwaAddSwt=1 : Constant  Value=LL_LKASWASyn_TrqSwaAddSwt  OutDataTypeStr=single
  LL_LKASWASyn_TrqSwaRateDiff=-0.2 : Constant  Value=LL_LKASWASyn_TrqSwaRateDiff  OutDataTypeStr=single
  LL_LKASWASyn_tiTrqSwaRtTime=0.2 : Constant  Value=LL_LKASWASyn_tiTrqSwaRtTime  OutDataTypeStr=single
  LL_LKASWASyn_tiTrqSwaTime=0.3 : Constant  Value=LL_LKASWASyn_tiTrqSwaTime  OutDataTypeStr=single
  LL_LSpdCompT_C=0.4 : Constant  Value=LL_LSpdCompT_C  OutDataTypeStr=single
  LL_NomTAhd_C=0.2 : Constant  Value=LL_NomTAhd_C  OutDataTypeStr=single
  LL_lStpLngth_C=5 : Constant  Value=LL_lStpLngth_C  OutDataTypeStr=single
  Switch{1..18,30..36,39..40,42..50,52..55} (40 alike) : Switch  Criteria=u2 ~= 0  OutDataTypeStr=single
  LKAClb : Outport
  wires:
  Bus Creator/1 -> LKAClb/1
  Switch8/1 -> Bus Creator/1  "LL_DvtPrvwT_C"
  Switch1/1 -> Bus Creator/2  "LL_DvtComp_C"
  Switch3/1 -> Bus Creator/3  "LL_HdAgPrvwT_C"
  Switch17/1 -> Bus Creator/12  "LL_CompSWA_C"
  Switch6/1 -> Bus Creator/7  "LL_HdAgExT_C"
  Switch7/1 -> Bus Creator/5  "LL_LAccMax_C"
  Switch4/1 -> Bus Creator/6  "LL_LAccRMax_C"
  Switch5/1 -> Bus Creator/8  "LL_LSpdCompT_C"
  Switch2/1 -> Bus Creator/4  "LL_CrvtPrvwT_C"
  Switch15/1 -> Bus Creator/10  "LL_lStpLngth_C"
  Switch10/1 -> Bus Creator/9  "LL_DesDvt_C"
  Switch12/1 -> Bus Creator/11  "LL_NomTAhd_C"
  LL_DvtPrvwT_C=0.45/1 -> Switch8/3
  Data Type Conversion8/1 -> Switch8/1, Switch8/2
  Data Type Conversion1/1 -> Switch1/2, Switch1/1
  LL_DvtComp_C=0/1 -> Switch1/3
  LL_CrvtPrvwT_C=0.45/1 -> Switch2/3
  Data Type Conversion16/1 -> Switch2/2, Switch2/1
  Data Type Conversion3/1 -> Switch3/2, Switch3/1
  LL_HdAgPrvwT_C=0.45/1 -> Switch3/3
  LL_HdAgExT_C=15/1 -> Switch6/3
  Data Type Conversion6/1 -> Switch6/2, Switch6/1
  Data Type Conversion13/1 -> Switch5/2, Switch5/1
  LL_LSpdCompT_C=0.4/1 -> Switch5/3
  LL_LAccRMax_C=5/1 -> Switch4/3
  Data Type Conversion10/1 -> Switch4/1, Switch4/2
  Data Type Conversion5/1 -> Switch7/2, Switch7/1
  LL_LAccMax_C=3/1 -> Switch7/3
  Data Type Conversion21/1 -> Switch15/2, Switch15/1
  Data Type Conversion23/1 -> Switch12/2, Switch12/1
  Data Type Conversion22/1 -> Switch10/2, Switch10/1
  Data Type Conversion2/1 -> Switch17/2, Switch17/1
  LL_DesDvt_C=0.2/1 -> Switch10/3
  LL_lStpLngth_C=5/1 -> Switch15/3
  LL_NomTAhd_C=0.2/1 -> Switch12/3
  LL_CompSWA_C=0/1 -> Switch17/3
  Bus Creator2/1 -> Bus Creator/13  "LL_TFCClb"
  Switch35/1 -> Bus Creator2/6  "LL_LFClb_TFC_facmGainLutGain2_C"
  Switch30/1 -> Bus Creator2/1  "LL_LFClb_TFC_facmKlat_C"
  Switch31/1 -> Bus Creator2/3  "LL_LFClb_TFC_vGainLutVehSpdLwr_C"
  Switch34/1 -> Bus Creator2/4  "LL_LFClb_TFC_vGainLutVehSpdUpr_C"
  Switch33/1 -> Bus Creator2/5  "LL_LFClb_TFC_facmGainLutGain1_C"
  Switch32/1 -> Bus Creator2/2  "LL_LFClb_TFC_tiKlatPrvwT_C"
  LL_LFClb_TFC_facmGainLutGain1_C=40/1 -> Switch33/3
  LL_LFClb_TFC_vGainLutVehSpdLwr_C=60/1 -> Switch31/3
  LL_LFClb_TFC_tiKlatPrvwT_C=1/1 -> Switch32/3
  Data Type Conversion11/1 -> Switch30/2, Switch30/1
  Data Type Conversion7/1 -> Switch33/2, Switch33/1
  Data Type Conversion4/1 -> Switch34/2, Switch34/1
  Data Type Conversion15/1 -> Switch32/2, Switch32/1
  Data Type Conversion17/1 -> Switch35/2, Switch35/1
  LL_LFClb_TFC_facmGainLutGain2_C=40/1 -> Switch35/3
  Data Type Conversion14/1 -> Switch31/2, Switch31/1
  LL_LFClb_TFC_vGainLutVehSpdUpr_C=120/1 -> Switch34/3
  LL_LFClb_TFC_facmKlat_C=-4.5/1 -> Switch30/3
  LL_LFClb_TFC_FfCtlRatio_C=1/1 -> Switch36/3
  Data Type Conversion18/1 -> Switch36/1, Switch36/2
  Switch36/1 -> Bus Creator2/7  "LL_LFClb_TFC_FfCtlRatio_C"
  Switch40/1 -> Bus Creator2/9  "LL_LFClb_TFC_facmIntegRatio"
  Switch39/1 -> Bus Creator2/8  "LL_LFClb_TFC_phiIntegCtlMaxSWA_C"
  LL_LFClb_TFC_phiIntegCtlMaxSWA_C=5/1 -> Switch39/3
  Data Type Conversion28/1 -> Switch39/1, Switch39/2
  LL_LFClb_TFC_facmIntegRatio=0.01/1 -> Switch40/3
  Data Type Conversion29/1 -> Switch40/1, Switch40/2
  Data Type Conversion31/1 -> Switch42/2, Switch42/1
  LL_LKASWASyn_TrqMax=1.5/1 -> Switch42/3
  LL_LKASWASyn_SWAaddMax=8/1 -> Switch43/3
  Data Type Conversion32/1 -> Switch43/1, Switch43/2
  Switch43/1 -> Bus Creator3/1  "LL_LKASWASyn_SWAaddMax"
  Switch42/1 -> Bus Creator3/2  "LL_LKASWASyn_TrqMax"
  Bus Creator3/1 -> Bus Creator/14  "LL_LKASWAClb"
  Switch44/1 -> Bus Creator4/4  "LL_LKAExPrcs_ExitC0Dvt"
  Switch45/1 -> Bus Creator4/3  "LL_LKAExPrcs_tiExitTime3"
  Data Type Conversion34/1 -> Switch45/2, Switch45/1
  LL_LKAExPrcs_tiExitTime3=0.2/1 -> Switch45/3
  LL_LKAExPrcs_ExitC0Dvt=0.01/1 -> Switch44/3
  Data Type Conversion33/1 -> Switch44/1, Switch44/2
  Bus Creator4/1 -> Bus Creator/15  "LL_LKAExPrcs"
  Data Type Conversion35/1 -> Switch46/2, Switch46/1
  LL_LKAExPrcs_ExitC0Swt=1/1 -> Switch46/3
  Switch46/1 -> Bus Creator4/5  "LL_LKAExPrcs_ExitC0Swt"
  Switch47/1 -> Bus Creator3/3  "LL_LKASWASyn_TrqSwaAddSwt"
  LL_LKASWASyn_TrqSwaAddSwt=1/1 -> Switch47/3
  Data Type Conversion47/1 -> Switch47/1, Switch47/2
  Data Type Conversion48/1 -> Switch48/2, Switch48/1
  LL_LFClb_TFC_DiffCtrlRatio=600/1 -> Switch48/3
  Switch48/1 -> Bus Creator2/11  "LL_LFClb_TFC_DiffCtrlRatio"
  Switch49/1 -> Bus Creator2/10  "LL_LFClb_TFC_DiffCtrlMaxSWA"
  LL_LFClb_TFC_DiffCtrlMaxSWA=20/1 -> Switch49/3
  Data Type Conversion49/1 -> Switch49/1, Switch49/2
  Data Type Conversion50/1 -> Switch50/2, Switch50/1
  LL_LKASWASyn_tiTrqSwaTime=0.3/1 -> Switch50/3
  Switch50/1 -> Bus Creator3/4  "LL_LKASWASyn_tiTrqSwaTime"
  Switch52/1 -> Bus Creator3/5  "LL_LKASWASyn_tiTrqSwaRtTime"
  LL_LKASWASyn_tiTrqSwaRtTime=0.2/1 -> Switch52/3
  Data Type Conversion52/1 -> Switch52/1, Switch52/2
  Data Type Conversion53/1 -> Switch53/2, Switch53/1
  LL_LKASWASyn_TrqSwaRateDiff=-0.2/1 -> Switch53/3
  Switch53/1 -> Bus Creator3/6  "LL_LKASWASyn_TrqSwaRateDiff"
  LL_LKAExPrcs_tiExitTime3=4/1 -> Switch54/3
  Data Type Conversion54/1 -> Switch54/1, Switch54/2
  Switch54/1 -> Bus Creator4/2  "LL_LKAExPrcs_tiExitTime2"
  Switch55/1 -> Bus Creator4/1  "LL_LKAExPrcs_tiExitTime1"
  Data Type Conversion55/1 -> Switch55/2, Switch55/1
  LL_LKAExPrcs_tiExitTime3=8/1 -> Switch55/3
  Switch9/1 -> Bus Creator2/12  "LL_LFClb_TFC_DiffCtlBalance"
  LL_LFClb_TFC_DiffCtlBalance=1.2/1 -> Switch9/3
  Data Type Conversion9/1 -> Switch9/1, Switch9/2
  [LLL_LKASWASyn_T2] -> Data Type Conversion24/1
  Switch16/1 -> Bus Creator3/10  "LL_LKASWASyn_T2"
  LL_LKASWASyn_T2=4/1 -> Switch16/3
  Data Type Conversion24/1 -> Switch16/1, Switch16/2
  Data Type Conversion20/1 -> Switch14/2, Switch14/1
  LL_LKASWASyn_M2=0.3/1 -> Switch14/3
  Switch14/1 -> Bus Creator3/9  "LL_LKASWASyn_M2"
  [LLL_LKASWASyn_M2] -> Data Type Conversion20/1
  [LLL_LKASWASyn_M1] -> Data Type Conversion19/1
  Switch13/1 -> Bus Creator3/8  "LL_LKASWASyn_M1"
  LL_LKASWASyn_M1=0.8/1 -> Switch13/3
  Data Type Conversion19/1 -> Switch13/1, Switch13/2
  Data Type Conversion12/1 -> Switch11/2, Switch11/1
  LL_LKASWASyn_M0=0.4/1 -> Switch11/3
  Switch11/1 -> Bus Creator3/7  "LL_LKASWASyn_M0"
  [LLL_LKASWASyn_M0] -> Data Type Conversion12/1
  Data Type Conversion25/1 -> Switch18/2, Switch18/1
  LL_LKASWASyn_M3K=0.2/1 -> Switch18/3
  Switch18/1 -> Bus Creator3/11  "LL_LKASWASyn_M3K"
  [LLL_LKASWASyn_M3K] -> Data Type Conversion25/1
